simulink model "Task1_3_ISSf_CBF"  (R2024b)
settings: Solver=ode45  StartTime=0.0  StopTime=30  MaxStep=0.01  RelTol=1e-3
InitFcn:
  | if ~exist('params','var'), params=System_Parameters(); end; if ~exist('simcfg','var'), simcfg=Simulink_Config(params); end;
undefined symbols (not defined in the file): params, simcfg
libraries: simulink_extras x1
settings Model: Creator=LAPTOPASADI  LastModifiedBy=LAPTOPASADI

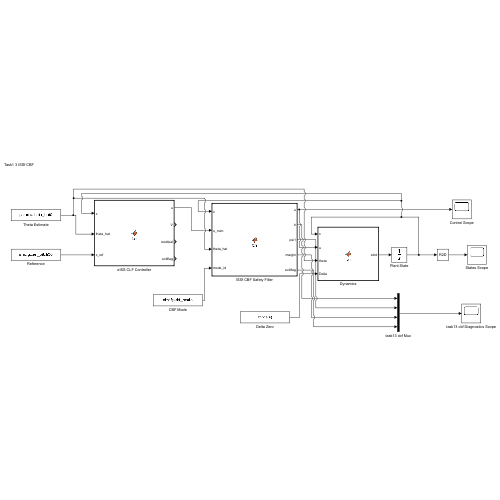
[thumbnail: Simulink's stored preview of the top-level diagram]
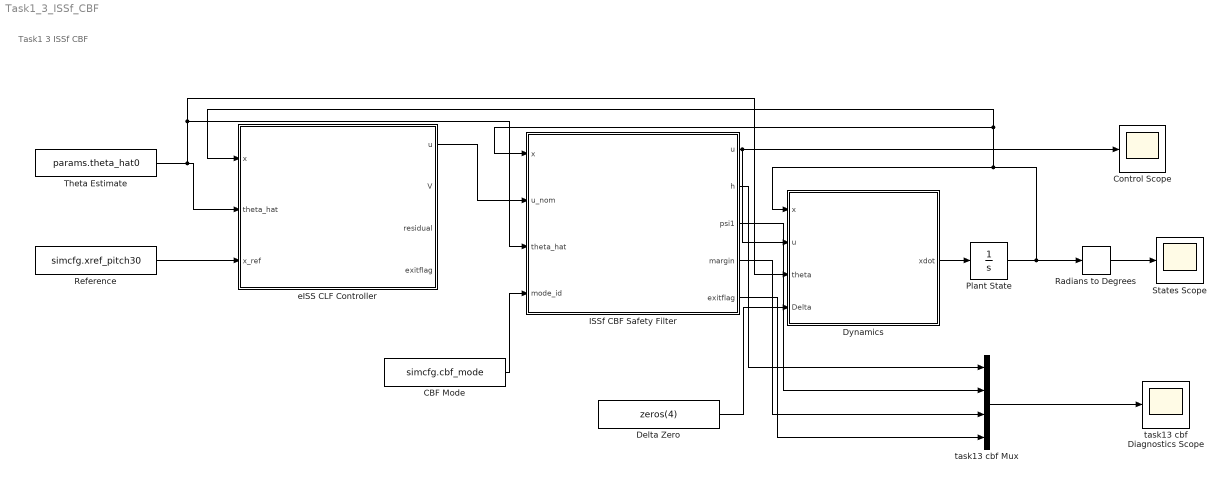
== system Task1_3_ISSf_CBF ==
  note: Task1 3 ISSf CBF
  CBF Mode : Constant  Value=simcfg.cbf_mode
  Control Scope : Scope
  Delta Zero : Constant  Value=zeros(4)
  Dynamics : MATLAB Function  TreatAsAtomicUnit=on
  ISSf CBF Safety Filter : MATLAB Function  TreatAsAtomicUnit=on
  Plant State : Integrator  InitialCondition=simcfg.x0_safe
  Radians to Degrees : simulink_extras/Transformations/Radians to Degrees
  Reference : Constant  Value=simcfg.xref_pitch30
  States Scope : Scope
  Theta Estimate : Constant  Value=params.theta_hat0
  eISS CLF Controller : MATLAB Function  TreatAsAtomicUnit=on
  task13 cbf Diagnostics Scope : Scope
  task13 cbf Mux : Mux
  wires:
  Plant State/1 -> eISS CLF Controller/1(x), ISSf CBF Safety Filter/1(x), Dynamics/1(x), Radians to Degrees/1
  Theta Estimate/1 -> eISS CLF Controller/2(theta_hat), ISSf CBF Safety Filter/3(theta_hat), Dynamics/3(theta)
  Reference/1 -> eISS CLF Controller/3(x_ref)
  eISS CLF Controller/1(u) -> ISSf CBF Safety Filter/2(u_nom)
  CBF Mode/1 -> ISSf CBF Safety Filter/4(mode_id)
  ISSf CBF Safety Filter/1(u) -> Dynamics/2(u), Control Scope/1
  Delta Zero/1 -> Dynamics/4(Delta)
  Dynamics/1(xdot) -> Plant State/1
  ISSf CBF Safety Filter/2(h) -> task13 cbf Mux/1
  ISSf CBF Safety Filter/3(psi1) -> task13 cbf Mux/2
  ISSf CBF Safety Filter/4(margin) -> task13 cbf Mux/3
  ISSf CBF Safety Filter/5(exitflag) -> task13 cbf Mux/4
  task13 cbf Mux/1 -> task13 cbf Diagnostics Scope/1
  Radians to Degrees/1 -> States Scope/1

== matlab function Task1_3_ISSf_CBF/ISSf CBF Safety Filter ==
  data: x input; u output; u_nom input; theta_hat input; mode_id input; h output; psi1 output; margin output; exitflag output
function [u,h,psi1,margin,exitflag] = fcn(x,u_nom,theta_hat,mode_id)
G = [0 0 40.75371832714017 8.6858779355964231;0 5.9859154929577469 0 0;0 0 2.4098880670272087 -9.893830239002293];
x=reshape(x,6,1);
u_nom=reshape(u_nom,4,1);
theta_hat=reshape(theta_hat,6,1);
theta_max = 0.3490658503988659;
alpha1 = 5;
alpha2 = 5;
kappa = 0.5;
lower = [-0.10000000000000001;-0.10000000000000001;-0.10000000000000001;-0.10000000000000001];
upper = [0.10000000000000001;0.10000000000000001;0.10000000000000001;0.10000000000000001];

[h,psi1,Lf,phi_h,Lg] = hocbf_terms(x,G,theta_max,alpha1);
iota = 0;
if mode_id >= 0.5
    iota = (phi_h'*phi_h)/kappa;
end
A = -Lg;
b = Lf+phi_h'*theta_hat+alpha2*psi1-iota;
[u,exitflag] = project_point(u_nom,A,b,lower,upper);
margin = Lf+phi_h'*theta_hat+Lg*u+alpha2*psi1-iota;
end

function [h,psi1,Lf,phi_h,Lg] = hocbf_terms(x,G,theta_max,alpha1)
phi=x(1); pitch=x(2); w=x(4:6);
[J,Jphi,Jpitch]=kinematics(phi,pitch);
rates=J*w; Jdot=Jphi*rates(1)+Jpitch*rates(2);
p=x(4); q=x(5); r=x(6);
Fw=[p*q,-q*r,0,0,0,-p; 0,0,p*r,-(p^2-r^2),0,-q; -q*r,0,0,0,p*q,-r];
J2=J(2,:); h=theta_max-pitch; hdot=-rates(2);
psi1=hdot+alpha1*h;
Lf=-Jdot(2,:)*w-alpha1*rates(2);
phi_h=(-J2*Fw)'; Lg=-J2*G;
end

function [J,Jphi,Jpitch] = kinematics(phi,pitch)
c=cos(phi); s=sin(phi); cp=cos(pitch);
if abs(cp)<1e-6, cp=sign(cp+eps)*1e-6; end
t=sin(pitch)/cp; sec=1/cp;
J=[1,s*t,c*t;0,c,-s;0,s*sec,c*sec];
Jphi=[0,c*t,-s*t;0,-s,-c;0,c*sec,-s*sec];
Jpitch=[0,s*sec^2,c*sec^2;0,0,0;0,s*sec*t,c*sec*t];
end

function [u,flag]=project_point(v,a,b,lower,upper)
tol=1e-10; u=min(max(v,lower),upper);
if a*u<=b+tol, flag=1; return; end
umin=upper; umin(a>=0)=lower(a>=0);
if a*umin>b+tol, u=umin; flag=-2; return; end
lo=0; hi=1;
while a*min(max(v-hi*a',lower),upper)>b
    hi=2*hi;
    if hi>1e12, u=umin; flag=-2; return; end
end
for k=1:80
    mid=0.5*(lo+hi); candidate=min(max(v-mid*a',lower),upper);
    if a*candidate>b, lo=mid; else, hi=mid; end
end
u=min(max(v-hi*a',lower),upper); flag=1;
end

== matlab function Task1_3_ISSf_CBF/eISS CLF Controller ==
  data: x input; u output; theta_hat input; x_ref input; V output; residual output; exitflag output
function [u,V,residual,exitflag] = fcn(x,theta_hat,x_ref)
P = [0.11250000000000002 0 0 0.012500000000000001 0 0;0 0.11250000000000002 0 0 0.012500000000000001 0;0 0 0.11250000000000002 0 0 0.012500000000000001;0.012500000000000001 0 0 0.015625 0 0;0 0.012500000000000001 0 0 0.015625 0;0 0 0.012500000000000001 0 0 0.015625];
G = [0 0 40.75371832714017 8.6858779355964231;0 5.9859154929577469 0 0;0 0 2.4098880670272087 -9.893830239002293];
x=reshape(x,6,1);
theta_hat=reshape(theta_hat,6,1);
x_ref=reshape(x_ref,6,1);
c_eiss = 0.5;
kappa = 10;
lower = [-0.10000000000000001;-0.10000000000000001;-0.10000000000000001;-0.10000000000000001];
upper = [0.10000000000000001;0.10000000000000001;0.10000000000000001;0.10000000000000001];

[V,omega,phiV,LgV] = clf_terms(x,x_ref,P,G);
iota = (phiV'*phiV)/kappa;
b = -c_eiss*V+iota-omega-phiV'*theta_hat;
[u,exitflag] = project_origin(LgV,b,lower,upper);
residual = omega+phiV'*theta_hat+LgV*u+c_eiss*V-iota;
end

function [V,omega,phiV,LgV] = clf_terms(x,x_ref,P,G)
phi = x(1); pitch = x(2); w = x(4:6);
[J,Jphi,Jpitch] = kinematics(phi,pitch);
rates = J*w;
Jdot = Jphi*rates(1)+Jpitch*rates(2);
eta = [x(1:3)-x_ref(1:3); rates];
p = x(4); q = x(5); r = x(6);
Fw = [p*q,-q*r,0,0,0,-p; 0,0,p*r,-(p^2-r^2),0,-q; -q*r,0,0,0,p*q,-r];
grad = 2*P*eta;
V = eta'*P*eta;
omega = grad(1:3)'*rates+grad(4:6)'*(Jdot*w);
phiV = (J*Fw)'*grad(4:6);
LgV = grad(4:6)'*(J*G);
end

function [J,Jphi,Jpitch] = kinematics(phi,pitch)
c = cos(phi); s = sin(phi); cp = cos(pitch);
if abs(cp)<1e-6, cp=sign(cp+eps)*1e-6; end
t = sin(pitch)/cp; sec = 1/cp;
J = [1,s*t,c*t; 0,c,-s; 0,s*sec,c*sec];
Jphi = [0,c*t,-s*t; 0,-s,-c; 0,c*sec,-s*sec];
Jpitch = [0,s*sec^2,c*sec^2; 0,0,0; 0,s*sec*t,c*sec*t];
end

function [u,flag] = project_origin(a,b,lower,upper)
tol = 1e-12;
u = min(max(zeros(4,1),lower),upper);
if a*u <= b+tol, flag=1; return; end
umin = upper; umin(a>=0)=lower(a>=0);
if a*umin > b+tol, u=umin; flag=-2; return; end
lo=0; hi=1;
while a*min(max(-hi*a',lower),upper) > b
    hi=2*hi;
    if hi>1e12, u=umin; flag=-2; return; end
end
for k=1:80
    mid=0.5*(lo+hi); candidate=min(max(-mid*a',lower),upper);
    if a*candidate>b, lo=mid; else, hi=mid; end
end
u=min(max(-hi*a',lower),upper); flag=1;
end

== matlab function Task1_3_ISSf_CBF/Dynamics ==
  data: x input; u input; xdot output; theta input; Delta input
function xdot = fcn(x,u,theta,Delta)
G = [0 0 40.75371832714017 8.6858779355964231;0 5.9859154929577469 0 0;0 0 2.4098880670272087 -9.893830239002293];
x=reshape(x,6,1);
u=reshape(u,4,1);
theta=reshape(theta,6,1);
Delta=reshape(Delta,4,4);

phi = x(1);
pitch = x(2);
p = x(4);
q = x(5);
r = x(6);

cphi = cos(phi);
sphi = sin(phi);
cpitch = cos(pitch);
if abs(cpitch) < 1e-6
    cpitch = sign(cpitch+eps)*1e-6;
end
tpitch = sin(pitch)/cpitch;

J = [1, sphi*tpitch, cphi*tpitch;
     0, cphi,         -sphi;
     0, sphi/cpitch,  cphi/cpitch];
f0 = [J*[p;q;r]; zeros(3,1)];
Fomega = [p*q, -q*r, 0, 0, 0, -p;
          0, 0, p*r, -(p^2-r^2), 0, -q;
          -q*r, 0, 0, 0, p*q, -r];
F = [zeros(3,6); Fomega];
g = [zeros(3,4); G];
xdot = f0+F*theta+g*(eye(4)+Delta)*u;
end
